simulink library "IOBlock_Library_TTC580"  (R2021a)
settings: Solver=ode45  StartTime=0.0  StopTime=10.0  RelTol=1e-3
PreLoadFcn:
  | addpath(genpath(fileparts(which('IOBlock_Library_TTC580'))));
  | %addpath(genpath(fileparts(which('IOBlock_Library_TTC580.mdl'))))
  | try
  | addpath(genpath([fileparts(which('IOBlock_Library_TTC580')),'\..\DBC_Importer']));
  | addpath(genpath([fileparts(which('IOBlock_Library_TTC580')),'\..\EEPROM_Importer']));
  | addpath(genpath([fileparts(which('IOBlock_Library_TTC580')),'\..\UserDoc']));
  | catch
  | warning('IOBlock_Library_TTC580: add path to DBC_Importer and EEPROM_Importer manually');
  | end
  | try
  | if exist('..\CustomPackage\scripts\OpenAllPackages.m','file')
  |      run('..\CustomPackage\scripts\OpenAllPackages.m'); %always available, ggf. empty
  | end
  | catch
  | warning('A problem occurred opening automatically the CustomPackage. Please open libraries manually');
  | end
  | try
  | set_param(0,'EditorSmartEditingHotParam','off');
  | catch
  | warning('Simlink preferences for ''Edit key parameter when adding new blocks'' needs to be unchecked manually');
  | end
undefined symbols (not defined in the file or in its folder): ADC_Absolute_10V, ADC_Absolute_32V, ADC_Absolute_5V, ADC_BoardTemp, ADC_ChannelInit, ADC_Current, ADC_Get, ADC_K15_, ADC_Ratiometric_10V, ADC_Ratiometric_5V, ADC_Resistive, ADC_SensorSupply, ADC_UBAT, bit_packing, bit_unpacking, CAN_ConfigMsg, compare2error, compare2FET_PROT_REENABLE, crc32_calc_intern, CRC32_EEPROM_Read, CRC32_EEPROM_Write, DIAG_EnterSafestate, DIAG_Status, DIAG_Status_internal, EEPROM_Mirror, EEPROM_Read, EEPROM_Read_OffsetIn, EEPROM_Read_Raw, EEPROM_Write, EEPROM_Write_OffsetIn, EEPROM_Write_Raw, EnterSafestate, FPU_Handler, Get_DI, Get_DI_VarThreshold, Get_K15_, Get_Pulse_Freq_Curr, Get_Pulse_Freq_Volt, Get_WakeUp, GetDateAndTime, IO_ADC_ResetProtection, IO_Blk_Lib_TTC500, IO_CAN_ReadMsg, IO_CAN_WriteMsg, IO_DI_Get, IO_DI_Init, IO_DI_Init_Var, IO_DO_GetCur, IO_DO_GetVoltage, IO_DO_Init, IO_DO_ResetProtection, IO_DO_Set, IO_Driver_GetSerialNumber, IO_Driver_GetVersionOfDriver, IO_Driver_GetVersionOfFPGA, IO_EEPROM_GetStatus, IO_EEPROM_Init, IO_EEPROM_Read_raw, IO_EEPROM_Write, IO_EEPROM_Write_OffsetIn ... (+73)
libraries: simulink x43
(part 7 of 18)

== system IOBlock_Library_TTC580/ADC Blocks TTC580 IOlib/ADC_Absolute_5V ==
  ADC_ChannelInit : Subsystem  LoadFcn=|  mask(ADC_ChannelInit_Code){SampleTime=-1, ttlib=IO_Blk_Lib_TTC500, ttDescription=ADC_ChannelInit, tt_iolib_version=0.19, adc_channel=adc_channel, adc_type=adc_type, range=range, pupd=pupd, sensor_supply=sensor_supply, safety_conf=NULL}
      | try
      | %
      | %Upgrade Information - standard BEGIN
      | new_color = 'blue';
      | new_ver = '0.19';
      | act_ver = get_param(gcb,'tt_iolib_version');
      | if not(strcmp(act_ver,new_ver))
      |     disp(['Upgrade block: ',gcb,char(10),'       Version: ',act_ver,' -> ',new_ver]);
      |     %switch - case for specific upgrade information e.g. additional parameter required 
      |     %Change appearance and version information
      |     set_param(gcb,'ForegroundColor',new_color);
      |     set_param(gcb,'tt_iolib_version',new_ver);
      | end
      | %Upgrade Information - standard END
      | catch
      | %Standard catch section BEGIN 
      | disp(' ');
      | disp('------------------------------------------------------------');
      | disp('An error occurred in a callback of the TTC580-BlockLib.');
      | disp(['Please check the parameters in the mask of ',gcb]);
      | disp('If you do not encounter any violations, then please '); 
      | disp('copy the following lines and report this to support@ttcontrol.com ');
      | disp('<< begin of error message dump >>');
      | disp(['Version of TTC580-BlockLib: ', get_param(gcb,'tt_iolib_version')]);
      | disp(get_param(gcb,'ttDescription'));
      | disp(gcb);
      | x=lasterror;disp(x.message);
      | disp(get_param(gcb,'MaskValues'));
      | disp(version);
      | disp(computer);
      | disp('<< end of error message dump >>');
      | disp('------------------------------------------------------------');
      | disp(' ');
      | %Standard catch section END
      | end
      mask help: Setup one ADC channel.
      mask init:
      | %
      settings: CopyFcn=%deleted
      mask Help: web(which('IO_ADC.h'))
      mask Callback adc_channel: %
      mask Callback adc_type: %
      mask Callback range: %
      mask Callback pupd: %
      mask Callback sensor_supply: %
      mask Callback safety_conf: %
  ADC_Get : Subsystem  LoadFcn=|  mask(ADC_Get_Code){SampleTime=-1, ttlib=IO_Blk_Lib_TTC500, ttDescription=ADC_Get, tt_iolib_version=0.19, adc_channel=adc_channel}
      | try
      | %
      | %Upgrade Information - standard BEGIN
      | new_color = 'blue';
      | new_ver = '0.19';
      | act_ver = get_param(gcb,'tt_iolib_version');
      | if not(strcmp(act_ver,new_ver))
      |     disp(['Upgrade block: ',gcb,char(10),'       Version: ',act_ver,' -> ',new_ver]);
      |     %switch - case for specific upgrade information e.g. additional parameter required 
      |     %Change appearance and version information
      |     set_param(gcb,'ForegroundColor',new_color);
      |     set_param(gcb,'tt_iolib_version',new_ver);
      | end
      | %Upgrade Information - standard END
      | catch
      | %Standard catch section BEGIN 
      | disp(' ');
      | disp('------------------------------------------------------------');
      | disp('An error occurred in a callback of the TTC580-BlockLib.');
      | disp(['Please check the parameters in the mask of ',gcb]);
      | disp('If you do not encounter any violations, then please '); 
      | disp('copy the following lines and report this to support@ttcontrol.com ');
      | disp('<< begin of error message dump >>');
      | disp(['Version of TTC580-BlockLib: ', get_param(gcb,'tt_iolib_version')]);
      | disp(get_param(gcb,'ttDescription'));
      | disp(gcb);
      | x=lasterror;disp(x.message);
      | disp(get_param(gcb,'MaskValues'));
      | disp(version);
      | disp(computer);
      | disp('<< end of error message dump >>');
      | disp('------------------------------------------------------------');
      | disp(' ');
      | %Standard catch section END
      | end
      mask help: Returns the value of the given ADC channel.
      mask init:
      | %
      settings: CopyFcn=%deleted
      mask Help: web(which('IO_ADC.h'))
      mask Callback adc_channel: %
  PWM_Init : Terminator
  PWM_Init1 : Terminator
  ErrorCode : Outport  VectorParamsAs1DForOutWhenUnconnected=off
  adc_value : Outport  Port=2  VectorParamsAs1DForOutWhenUnconnected=off
  wires:
  ADC_ChannelInit/1(ErrorCode) -> PWM_Init/1
  ADC_Get/3(fresh) -> PWM_Init1/1
  ADC_Get/1(ErrorCode) -> ErrorCode/1
  ADC_Get/2(adc_value) -> adc_value/1

== system IOBlock_Library_TTC580/ADC Blocks TTC580 IOlib/ADC_BoardTemp ==
  ADC_ChannelInit : Subsystem  LoadFcn=|  mask(ADC_ChannelInit_Code){SampleTime=-1, ttlib=IO_Blk_Lib_TTC500, ttDescription=ADC_ChannelInit, tt_iolib_version=0.19, adc_channel=adc_channel, adc_type=adc_type, range=range, pupd=pupd, sensor_supply=sensor_supply, safety_conf=NULL}
      | try
      | %
      | %Upgrade Information - standard BEGIN
      | new_color = 'blue';
      | new_ver = '0.19';
      | act_ver = get_param(gcb,'tt_iolib_version');
      | if not(strcmp(act_ver,new_ver))
      |     disp(['Upgrade block: ',gcb,char(10),'       Version: ',act_ver,' -> ',new_ver]);
      |     %switch - case for specific upgrade information e.g. additional parameter required 
      |     %Change appearance and version information
      |     set_param(gcb,'ForegroundColor',new_color);
      |     set_param(gcb,'tt_iolib_version',new_ver);
      | end
      | %Upgrade Information - standard END
      | catch
      | %Standard catch section BEGIN 
      | disp(' ');
      | disp('------------------------------------------------------------');
      | disp('An error occurred in a callback of the TTC580-BlockLib.');
      | disp(['Please check the parameters in the mask of ',gcb]);
      | disp('If you do not encounter any violations, then please '); 
      | disp('copy the following lines and report this to support@ttcontrol.com ');
      | disp('<< begin of error message dump >>');
      | disp(['Version of TTC580-BlockLib: ', get_param(gcb,'tt_iolib_version')]);
      | disp(get_param(gcb,'ttDescription'));
      | disp(gcb);
      | x=lasterror;disp(x.message);
      | disp(get_param(gcb,'MaskValues'));
      | disp(version);
      | disp(computer);
      | disp('<< end of error message dump >>');
      | disp('------------------------------------------------------------');
      | disp(' ');
      | %Standard catch section END
      | end
      mask help: Setup one ADC channel.
      mask init:
      | %
      settings: CopyFcn=%deleted
      mask Help: web(which('IO_ADC.h'))
      mask Callback adc_channel: %
      mask Callback adc_type: %
      mask Callback range: %
      mask Callback pupd: %
      mask Callback sensor_supply: %
      mask Callback safety_conf: %
  ADC_Get : Subsystem  LoadFcn=|  mask(ADC_Get_Code){SampleTime=-1, ttlib=IO_Blk_Lib_TTC500, ttDescription=ADC_Get, tt_iolib_version=0.19, adc_channel=adc_channel}
      | try
      | %
      | %Upgrade Information - standard BEGIN
      | new_color = 'blue';
      | new_ver = '0.19';
      | act_ver = get_param(gcb,'tt_iolib_version');
      | if not(strcmp(act_ver,new_ver))
      |     disp(['Upgrade block: ',gcb,char(10),'       Version: ',act_ver,' -> ',new_ver]);
      |     %switch - case for specific upgrade information e.g. additional parameter required 
      |     %Change appearance and version information
      |     set_param(gcb,'ForegroundColor',new_color);
      |     set_param(gcb,'tt_iolib_version',new_ver);
      | end
      | %Upgrade Information - standard END
      | catch
      | %Standard catch section BEGIN 
      | disp(' ');
      | disp('------------------------------------------------------------');
      | disp('An error occurred in a callback of the TTC580-BlockLib.');
      | disp(['Please check the parameters in the mask of ',gcb]);
      | disp('If you do not encounter any violations, then please '); 
      | disp('copy the following lines and report this to support@ttcontrol.com ');
      | disp('<< begin of error message dump >>');
      | disp(['Version of TTC580-BlockLib: ', get_param(gcb,'tt_iolib_version')]);
      | disp(get_param(gcb,'ttDescription'));
      | disp(gcb);
      | x=lasterror;disp(x.message);
      | disp(get_param(gcb,'MaskValues'));
      | disp(version);
      | disp(computer);
      | disp('<< end of error message dump >>');
      | disp('------------------------------------------------------------');
      | disp(' ');
      | %Standard catch section END
      | end
      mask help: Returns the value of the given ADC channel.
      mask init:
      | %
      settings: CopyFcn=%deleted
      mask Help: web(which('IO_ADC.h'))
      mask Callback adc_channel: %
  Add : Sum  Inputs=+-
  Constant : Constant  Value=10000  OutDataTypeStr=int32
  Constant1 : Constant  Value=100  OutDataTypeStr=int32
  Data Type Conversion : DataTypeConversion  OutDataTypeStr=int32
  Divide : Product  Inputs=*/
  PWM_Init : Terminator
  PWM_Init1 : Terminator
  ErrorCode : Outport  VectorParamsAs1DForOutWhenUnconnected=off
  Temperature : Outport  Port=2  VectorParamsAs1DForOutWhenUnconnected=off
  wires:
  ADC_ChannelInit/1(ErrorCode) -> PWM_Init/1
  ADC_Get/3(fresh) -> PWM_Init1/1
  ADC_Get/1(ErrorCode) -> ErrorCode/1
  ADC_Get/2(adc_value) -> Data Type Conversion/1
  Data Type Conversion/1 -> Add/1
  Constant/1 -> Add/2
  Add/1 -> Divide/1
  Constant1/1 -> Divide/2
  Divide/1 -> Temperature/1

== system IOBlock_Library_TTC580/ADC Blocks TTC580 IOlib/ADC_Current ==
  ADC_ChannelInit : Subsystem  LoadFcn=|  mask(ADC_ChannelInit_Code){SampleTime=-1, ttlib=IO_Blk_Lib_TTC500, ttDescription=ADC_ChannelInit, tt_iolib_version=0.19, adc_channel=adc_channel, adc_type=adc_type, range=range, pupd=pupd, sensor_supply=sensor_supply, safety_conf=NULL}
      | try
      | %
      | %Upgrade Information - standard BEGIN
      | new_color = 'blue';
      | new_ver = '0.19';
      | act_ver = get_param(gcb,'tt_iolib_version');
      | if not(strcmp(act_ver,new_ver))
      |     disp(['Upgrade block: ',gcb,char(10),'       Version: ',act_ver,' -> ',new_ver]);
      |     %switch - case for specific upgrade information e.g. additional parameter required 
      |     %Change appearance and version information
      |     set_param(gcb,'ForegroundColor',new_color);
      |     set_param(gcb,'tt_iolib_version',new_ver);
      | end
      | %Upgrade Information - standard END
      | catch
      | %Standard catch section BEGIN 
      | disp(' ');
      | disp('------------------------------------------------------------');
      | disp('An error occurred in a callback of the TTC580-BlockLib.');
      | disp(['Please check the parameters in the mask of ',gcb]);
      | disp('If you do not encounter any violations, then please '); 
      | disp('copy the following lines and report this to support@ttcontrol.com ');
      | disp('<< begin of error message dump >>');
      | disp(['Version of TTC580-BlockLib: ', get_param(gcb,'tt_iolib_version')]);
      | disp(get_param(gcb,'ttDescription'));
      | disp(gcb);
      | x=lasterror;disp(x.message);
      | disp(get_param(gcb,'MaskValues'));
      | disp(version);
      | disp(computer);
      | disp('<< end of error message dump >>');
      | disp('------------------------------------------------------------');
      | disp(' ');
      | %Standard catch section END
      | end
      mask help: Setup one ADC channel.
      mask init:
      | %
      settings: CopyFcn=%deleted
      mask Help: web(which('IO_ADC.h'))
      mask Callback adc_channel: %
      mask Callback adc_type: %
      mask Callback range: %
      mask Callback pupd: %
      mask Callback sensor_supply: %
      mask Callback safety_conf: %
  ADC_Get : Subsystem  LoadFcn=|  mask(ADC_Get_Code){SampleTime=-1, ttlib=IO_Blk_Lib_TTC500, ttDescription=ADC_Get, tt_iolib_version=0.19, adc_channel=adc_channel}
      | try
      | %
      | %Upgrade Information - standard BEGIN
      | new_color = 'blue';
      | new_ver = '0.19';
      | act_ver = get_param(gcb,'tt_iolib_version');
      | if not(strcmp(act_ver,new_ver))
      |     disp(['Upgrade block: ',gcb,char(10),'       Version: ',act_ver,' -> ',new_ver]);
      |     %switch - case for specific upgrade information e.g. additional parameter required 
      |     %Change appearance and version information
      |     set_param(gcb,'ForegroundColor',new_color);
      |     set_param(gcb,'tt_iolib_version',new_ver);
      | end
      | %Upgrade Information - standard END
      | catch
      | %Standard catch section BEGIN 
      | disp(' ');
      | disp('------------------------------------------------------------');
      | disp('An error occurred in a callback of the TTC580-BlockLib.');
      | disp(['Please check the parameters in the mask of ',gcb]);
      | disp('If you do not encounter any violations, then please '); 
      | disp('copy the following lines and report this to support@ttcontrol.com ');
      | disp('<< begin of error message dump >>');
      | disp(['Version of TTC580-BlockLib: ', get_param(gcb,'tt_iolib_version')]);
      | disp(get_param(gcb,'ttDescription'));
      | disp(gcb);
      | x=lasterror;disp(x.message);
      | disp(get_param(gcb,'MaskValues'));
      | disp(version);
      | disp(computer);
      | disp('<< end of error message dump >>');
      | disp('------------------------------------------------------------');
      | disp(' ');
      | %Standard catch section END
      | end
      mask help: Returns the value of the given ADC channel.
      mask init:
      | %
      settings: CopyFcn=%deleted
      mask Help: web(which('IO_ADC.h'))
      mask Callback adc_channel: %
  IO_ADC_ResetProtection : Subsystem  LoadFcn=|  mask(IO_ADC_ResetProtection_Code){SampleTime=-1, ttlib=IO_Blk_Lib_TTC500, ttDescription=IO_ADC_ResetProtection, tt_iolib_version=0.19, adc_channel=adc_channel}
      | try
      | %
      | %Upgrade Information - standard BEGIN
      | new_color = 'blue';
      | new_ver = '0.19';
      | act_ver = get_param(gcb,'tt_iolib_version');
      | if not(strcmp(act_ver,new_ver))
      |     disp(['Upgrade block: ',gcb,char(10),'       Version: ',act_ver,' -> ',new_ver]);
      |     %switch - case for specific upgrade information e.g. additional parameter required 
      |     %Change appearance and version information
      |     set_param(gcb,'ForegroundColor',new_color);
      |     set_param(gcb,'tt_iolib_version',new_ver);
      | end
      | %Upgrade Information - standard END
      | catch
      | %Standard catch section BEGIN 
      | disp(' ');
      | disp('------------------------------------------------------------');
      | disp('An error occurred in a callback of the TTC580-BlockLib.');
      | disp(['Please check the parameters in the mask of ',gcb]);
      | disp('If you do not encounter any violations, then please '); 
      | disp('copy the following lines and report this to support@ttcontrol.com ');
      | disp('<< begin of error message dump >>');
      | disp(['Version of TTC580-BlockLib: ', get_param(gcb,'tt_iolib_version')]);
      | disp(get_param(gcb,'ttDescription'));
      | disp(gcb);
      | x=lasterror;disp(x.message);
      | disp(get_param(gcb,'MaskValues'));
      | disp(version);
      | disp(computer);
      | disp('<< end of error message dump >>');
      | disp('------------------------------------------------------------');
      | disp(' ');
      | %Standard catch section END
      | end
      mask help: Reset the FET protection for an ADC channel.
      mask init:
      | %
      settings: CopyFcn=%deleted
      mask Help: web(which('IO_ADC.h'))
      mask Callback adc_channel: %
  PWM_Init : Terminator
  PWM_Init1 : Terminator
  Terminator1 : Terminator
  Terminator3 : Terminator
  compare2FET_PROT_REENABLE : Subsystem  LoadFcn=|  mask(compare2FET_PROT_REENABLE_Code){SampleTime=-1, ttlib=IO_Blk_Lib_TTC500, ttDescription=compare2FET_PROT_REENABLE, tt_iolib_version=0.19, define=IO_E_FET_PROT_REENABLE}
      | try
      | %
      | %Upgrade Information - standard BEGIN
      | new_color = 'blue';
      | new_ver = '0.19';
      | act_ver = get_param(gcb,'tt_iolib_version');
      | if not(strcmp(act_ver,new_ver))
      |     disp(['Upgrade block: ',gcb,char(10),'       Version: ',act_ver,' -> ',new_ver]);
      |     %switch - case for specific upgrade information e.g. additional parameter required 
      |     %Change appearance and version information
      |     set_param(gcb,'ForegroundColor',new_color);
      |     set_param(gcb,'tt_iolib_version',new_ver);
      | end
      | %Upgrade Information - standard END
      | catch
      | %Standard catch section BEGIN 
      | disp(' ');
      | disp('------------------------------------------------------------');
      | disp('An error occurred in a callback of the TTC580-BlockLib.');
      | disp(['Please check the parameters in the mask of ',gcb]);
      | disp('If you do not encounter any violations, then please '); 
      | disp('copy the following lines and report this to support@ttcontrol.com ');
      | disp('<< begin of error message dump >>');
      | disp(['Version of TTC580-BlockLib: ', get_param(gcb,'tt_iolib_version')]);
      | disp(get_param(gcb,'ttDescription'));
      | disp(gcb);
      | x=lasterror;disp(x.message);
      | disp(get_param(gcb,'MaskValues'));
      | disp(version);
      | disp(computer);
      | disp('<< end of error message dump >>');
      | disp('------------------------------------------------------------');
      | disp(' ');
      | %Standard catch section END
      | end
      mask help: The ErrorCode that is output from an I/O-Block is compared against IO_E_FET_PROT_REENABLE.
      mask init:
      | %
      settings: CopyFcn=%deleted
      mask Help: web(which('~.h'))
      mask Callback define: %
  ErrorCode : Outport  VectorParamsAs1DForOutWhenUnconnected=off
  adc_value : Outport  Port=2  VectorParamsAs1DForOutWhenUnconnected=off
  wires:
  ADC_ChannelInit/1(ErrorCode) -> PWM_Init/1
  ADC_Get/3(fresh) -> PWM_Init1/1
  ADC_Get/1(ErrorCode) -> ErrorCode/1, compare2FET_PROT_REENABLE/1(Errorcode)
  ADC_Get/2(adc_value) -> adc_value/1
  IO_ADC_ResetProtection/1(ErrorCode) -> Terminator3/1
  IO_ADC_ResetProtection/2(reset_cnt) -> Terminator1/1
  compare2FET_PROT_REENABLE/1(b_compare) -> IO_ADC_ResetProtection/Trigger

== system IOBlock_Library_TTC580/ADC Blocks TTC580 IOlib/ADC_K15_ ==
  ADC_ChannelInit : Subsystem  LoadFcn=|  mask(ADC_ChannelInit_Code){SampleTime=-1, ttlib=IO_Blk_Lib_TTC500, ttDescription=ADC_ChannelInit, tt_iolib_version=0.19, adc_channel=adc_channel, adc_type=adc_type, range=range, pupd=pupd, sensor_supply=sensor_supply, safety_conf=NULL}
      | try
      | %
      | %Upgrade Information - standard BEGIN
      | new_color = 'blue';
      | new_ver = '0.19';
      | act_ver = get_param(gcb,'tt_iolib_version');
      | if not(strcmp(act_ver,new_ver))
      |     disp(['Upgrade block: ',gcb,char(10),'       Version: ',act_ver,' -> ',new_ver]);
      |     %switch - case for specific upgrade information e.g. additional parameter required 
      |     %Change appearance and version information
      |     set_param(gcb,'ForegroundColor',new_color);
      |     set_param(gcb,'tt_iolib_version',new_ver);
      | end
      | %Upgrade Information - standard END
      | catch
      | %Standard catch section BEGIN 
      | disp(' ');
      | disp('------------------------------------------------------------');
      | disp('An error occurred in a callback of the TTC580-BlockLib.');
      | disp(['Please check the parameters in the mask of ',gcb]);
      | disp('If you do not encounter any violations, then please '); 
      | disp('copy the following lines and report this to support@ttcontrol.com ');
      | disp('<< begin of error message dump >>');
      | disp(['Version of TTC580-BlockLib: ', get_param(gcb,'tt_iolib_version')]);
      | disp(get_param(gcb,'ttDescription'));
      | disp(gcb);
      | x=lasterror;disp(x.message);
      | disp(get_param(gcb,'MaskValues'));
      | disp(version);
      | disp(computer);
      | disp('<< end of error message dump >>');
      | disp('------------------------------------------------------------');
      | disp(' ');
      | %Standard catch section END
      | end
      mask help: Setup one ADC channel.
      mask init:
      | %
      settings: CopyFcn=%deleted
      mask Help: web(which('IO_ADC.h'))
      mask Callback adc_channel: %
      mask Callback adc_type: %
      mask Callback range: %
      mask Callback pupd: %
      mask Callback sensor_supply: %
      mask Callback safety_conf: %
  ADC_Get : Subsystem  LoadFcn=|  mask(ADC_Get_Code){SampleTime=-1, ttlib=IO_Blk_Lib_TTC500, ttDescription=ADC_Get, tt_iolib_version=0.19, adc_channel=adc_channel}
      | try
      | %
      | %Upgrade Information - standard BEGIN
      | new_color = 'blue';
      | new_ver = '0.19';
      | act_ver = get_param(gcb,'tt_iolib_version');
      | if not(strcmp(act_ver,new_ver))
      |     disp(['Upgrade block: ',gcb,char(10),'       Version: ',act_ver,' -> ',new_ver]);
      |     %switch - case for specific upgrade information e.g. additional parameter required 
      |     %Change appearance and version information
      |     set_param(gcb,'ForegroundColor',new_color);
      |     set_param(gcb,'tt_iolib_version',new_ver);
      | end
      | %Upgrade Information - standard END
      | catch
      | %Standard catch section BEGIN 
      | disp(' ');
      | disp('------------------------------------------------------------');
      | disp('An error occurred in a callback of the TTC580-BlockLib.');
      | disp(['Please check the parameters in the mask of ',gcb]);
      | disp('If you do not encounter any violations, then please '); 
      | disp('copy the following lines and report this to support@ttcontrol.com ');
      | disp('<< begin of error message dump >>');
      | disp(['Version of TTC580-BlockLib: ', get_param(gcb,'tt_iolib_version')]);
      | disp(get_param(gcb,'ttDescription'));
      | disp(gcb);
      | x=lasterror;disp(x.message);
      | disp(get_param(gcb,'MaskValues'));
      | disp(version);
      | disp(computer);
      | disp('<< end of error message dump >>');
      | disp('------------------------------------------------------------');
      | disp(' ');
      | %Standard catch section END
      | end
      mask help: Returns the value of the given ADC channel.
      mask init:
      | %
      settings: CopyFcn=%deleted
      mask Help: web(which('IO_ADC.h'))
      mask Callback adc_channel: %
  PWM_Init : Terminator
  PWM_Init1 : Terminator
  ErrorCode : Outport  VectorParamsAs1DForOutWhenUnconnected=off
  adc_value : Outport  Port=2  VectorParamsAs1DForOutWhenUnconnected=off
  wires:
  ADC_Get/3(fresh) -> PWM_Init1/1
  ADC_Get/2(adc_value) -> adc_value/1
  ADC_Get/1(ErrorCode) -> ErrorCode/1
  ADC_ChannelInit/1(ErrorCode) -> PWM_Init/1

== system IOBlock_Library_TTC580/ADC Blocks TTC580 IOlib/ADC_Ratiometric_10V ==
  ADC_ChannelInit : Subsystem  LoadFcn=|  mask(ADC_ChannelInit_Code){SampleTime=-1, ttlib=IO_Blk_Lib_TTC500, ttDescription=ADC_ChannelInit, tt_iolib_version=0.19, adc_channel=adc_channel, adc_type=adc_type, range=range, pupd=pupd, sensor_supply=sensor_supply, safety_conf=NULL}
      | try
      | %
      | %Upgrade Information - standard BEGIN
      | new_color = 'blue';
      | new_ver = '0.19';
      | act_ver = get_param(gcb,'tt_iolib_version');
      | if not(strcmp(act_ver,new_ver))
      |     disp(['Upgrade block: ',gcb,char(10),'       Version: ',act_ver,' -> ',new_ver]);
      |     %switch - case for specific upgrade information e.g. additional parameter required 
      |     %Change appearance and version information
      |     set_param(gcb,'ForegroundColor',new_color);
      |     set_param(gcb,'tt_iolib_version',new_ver);
      | end
      | %Upgrade Information - standard END
      | catch
      | %Standard catch section BEGIN 
      | disp(' ');
      | disp('------------------------------------------------------------');
      | disp('An error occurred in a callback of the TTC580-BlockLib.');
      | disp(['Please check the parameters in the mask of ',gcb]);
      | disp('If you do not encounter any violations, then please '); 
      | disp('copy the following lines and report this to support@ttcontrol.com ');
      | disp('<< begin of error message dump >>');
      | disp(['Version of TTC580-BlockLib: ', get_param(gcb,'tt_iolib_version')]);
      | disp(get_param(gcb,'ttDescription'));
      | disp(gcb);
      | x=lasterror;disp(x.message);
      | disp(get_param(gcb,'MaskValues'));
      | disp(version);
      | disp(computer);
      | disp('<< end of error message dump >>');
      | disp('------------------------------------------------------------');
      | disp(' ');
      | %Standard catch section END
      | end
      mask help: Setup one ADC channel.
      mask init:
      | %
      settings: CopyFcn=%deleted
      mask Help: web(which('IO_ADC.h'))
      mask Callback adc_channel: %
      mask Callback adc_type: %
      mask Callback range: %
      mask Callback pupd: %
      mask Callback sensor_supply: %
      mask Callback safety_conf: %
  ADC_Get : Subsystem  LoadFcn=|  mask(ADC_Get_Code){SampleTime=-1, ttlib=IO_Blk_Lib_TTC500, ttDescription=ADC_Get, tt_iolib_version=0.19, adc_channel=adc_channel}
      | try
      | %
      | %Upgrade Information - standard BEGIN
      | new_color = 'blue';
      | new_ver = '0.19';
      | act_ver = get_param(gcb,'tt_iolib_version');
      | if not(strcmp(act_ver,new_ver))
      |     disp(['Upgrade block: ',gcb,char(10),'       Version: ',act_ver,' -> ',new_ver]);
      |     %switch - case for specific upgrade information e.g. additional parameter required 
      |     %Change appearance and version information
      |     set_param(gcb,'ForegroundColor',new_color);
      |     set_param(gcb,'tt_iolib_version',new_ver);
      | end
      | %Upgrade Information - standard END
      | catch
      | %Standard catch section BEGIN 
      | disp(' ');
      | disp('------------------------------------------------------------');
      | disp('An error occurred in a callback of the TTC580-BlockLib.');
      | disp(['Please check the parameters in the mask of ',gcb]);
      | disp('If you do not encounter any violations, then please '); 
      | disp('copy the following lines and report this to support@ttcontrol.com ');
      | disp('<< begin of error message dump >>');
      | disp(['Version of TTC580-BlockLib: ', get_param(gcb,'tt_iolib_version')]);
      | disp(get_param(gcb,'ttDescription'));
      | disp(gcb);
      | x=lasterror;disp(x.message);
      | disp(get_param(gcb,'MaskValues'));
      | disp(version);
      | disp(computer);
      | disp('<< end of error message dump >>');
      | disp('------------------------------------------------------------');
      | disp(' ');
      | %Standard catch section END
      | end
      mask help: Returns the value of the given ADC channel.
      mask init:
      | %
      settings: CopyFcn=%deleted
      mask Help: web(which('IO_ADC.h'))
      mask Callback adc_channel: %
  POWER_Set_Init : Subsystem  LoadFcn=|  mask(POWER_Set_Init_Code){SampleTime=-1, ttlib=IO_Blk_Lib_TTC500, ttDescription=POWER_Set_Init, tt_iolib_version=0.19, pin=sensor_supply, mode=volt_sensor_supply}
      | try
      | %
      | %Upgrade Information - standard BEGIN
      | new_color = 'blue';
      | new_ver = '0.19';
      | act_ver = get_param(gcb,'tt_iolib_version');
      | if not(strcmp(act_ver,new_ver))
      |     disp(['Upgrade block: ',gcb,char(10),'       Version: ',act_ver,' -> ',new_ver]);
      |     %switch - case for specific upgrade information e.g. additional parameter required 
      |     %Change appearance and version information
      |     set_param(gcb,'ForegroundColor',new_color);
      |     set_param(gcb,'tt_iolib_version',new_ver);
      | end
      | %Upgrade Information - standard END
      | catch
      | %Standard catch section BEGIN 
      | disp(' ');
      | disp('------------------------------------------------------------');
      | disp('An error occurred in a callback of the TTC580-BlockLib.');
      | disp(['Please check the parameters in the mask of ',gcb]);
      | disp('If you do not encounter any violations, then please '); 
      | disp('copy the following lines and report this to support@ttcontrol.com ');
      | disp('<< begin of error message dump >>');
      | disp(['Version of TTC580-BlockLib: ', get_param(gcb,'tt_iolib_version')]);
      | disp(get_param(gcb,'ttDescription'));
      | disp(gcb);
      | x=lasterror;disp(x.message);
      | disp(get_param(gcb,'MaskValues'));
      | disp(version);
      | disp(computer);
      | disp('<< end of error message dump >>');
      | disp('------------------------------------------------------------');
      | disp(' ');
      | %Standard catch section END
      | end
      mask help: Sets a certain mode of the Power IC.
      mask init:
      | %
      settings: CopyFcn=%deleted
      mask Help: web(which('IO_POWER.h'))
      mask Callback pin: %
      mask Callback mode: %
  PWM_Init : Terminator
  PWM_Init1 : Terminator
  PWM_Init2 : Terminator
  ErrorCode : Outport  VectorParamsAs1DForOutWhenUnconnected=off
  adc_value : Outport  Port=2  VectorParamsAs1DForOutWhenUnconnected=off
  wires:
  ADC_ChannelInit/1(ErrorCode) -> PWM_Init/1
  ADC_Get/3(fresh) -> PWM_Init1/1
  ADC_Get/1(ErrorCode) -> ErrorCode/1
  ADC_Get/2(adc_value) -> adc_value/1
  POWER_Set_Init/1(ErrorCode) -> PWM_Init2/1

== system IOBlock_Library_TTC580/ADC Blocks TTC580 IOlib/ADC_Ratiometric_5V ==
  ADC_ChannelInit : Subsystem  LoadFcn=|  mask(ADC_ChannelInit_Code){SampleTime=-1, ttlib=IO_Blk_Lib_TTC500, ttDescription=ADC_ChannelInit, tt_iolib_version=0.19, adc_channel=adc_channel, adc_type=adc_type, range=range, pupd=pupd, sensor_supply=sensor_supply, safety_conf=NULL}
      | try
      | %
      | %Upgrade Information - standard BEGIN
      | new_color = 'blue';
      | new_ver = '0.19';
      | act_ver = get_param(gcb,'tt_iolib_version');
      | if not(strcmp(act_ver,new_ver))
      |     disp(['Upgrade block: ',gcb,char(10),'       Version: ',act_ver,' -> ',new_ver]);
      |     %switch - case for specific upgrade information e.g. additional parameter required 
      |     %Change appearance and version information
      |     set_param(gcb,'ForegroundColor',new_color);
      |     set_param(gcb,'tt_iolib_version',new_ver);
      | end
      | %Upgrade Information - standard END
      | catch
      | %Standard catch section BEGIN 
      | disp(' ');
      | disp('------------------------------------------------------------');
      | disp('An error occurred in a callback of the TTC580-BlockLib.');
      | disp(['Please check the parameters in the mask of ',gcb]);
      | disp('If you do not encounter any violations, then please '); 
      | disp('copy the following lines and report this to support@ttcontrol.com ');
      | disp('<< begin of error message dump >>');
      | disp(['Version of TTC580-BlockLib: ', get_param(gcb,'tt_iolib_version')]);
      | disp(get_param(gcb,'ttDescription'));
      | disp(gcb);
      | x=lasterror;disp(x.message);
      | disp(get_param(gcb,'MaskValues'));
      | disp(version);
      | disp(computer);
      | disp('<< end of error message dump >>');
      | disp('------------------------------------------------------------');
      | disp(' ');
      | %Standard catch section END
      | end
      mask help: Setup one ADC channel.
      mask init:
      | %
      settings: CopyFcn=%deleted
      mask Help: web(which('IO_ADC.h'))
      mask Callback adc_channel: %
      mask Callback adc_type: %
      mask Callback range: %
      mask Callback pupd: %
      mask Callback sensor_supply: %
      mask Callback safety_conf: %
  ADC_Get : Subsystem  LoadFcn=|  mask(ADC_Get_Code){SampleTime=-1, ttlib=IO_Blk_Lib_TTC500, ttDescription=ADC_Get, tt_iolib_version=0.19, adc_channel=adc_channel}
      | try
      | %
      | %Upgrade Information - standard BEGIN
      | new_color = 'blue';
      | new_ver = '0.19';
      | act_ver = get_param(gcb,'tt_iolib_version');
      | if not(strcmp(act_ver,new_ver))
      |     disp(['Upgrade block: ',gcb,char(10),'       Version: ',act_ver,' -> ',new_ver]);
      |     %switch - case for specific upgrade information e.g. additional parameter required 
      |     %Change appearance and version information
      |     set_param(gcb,'ForegroundColor',new_color);
      |     set_param(gcb,'tt_iolib_version',new_ver);
      | end
      | %Upgrade Information - standard END
      | catch
      | %Standard catch section BEGIN 
      | disp(' ');
      | disp('------------------------------------------------------------');
      | disp('An error occurred in a callback of the TTC580-BlockLib.');
      | disp(['Please check the parameters in the mask of ',gcb]);
      | disp('If you do not encounter any violations, then please '); 
      | disp('copy the following lines and report this to support@ttcontrol.com ');
      | disp('<< begin of error message dump >>');
      | disp(['Version of TTC580-BlockLib: ', get_param(gcb,'tt_iolib_version')]);
      | disp(get_param(gcb,'ttDescription'));
      | disp(gcb);
      | x=lasterror;disp(x.message);
      | disp(get_param(gcb,'MaskValues'));
      | disp(version);
      | disp(computer);
      | disp('<< end of error message dump >>');
      | disp('------------------------------------------------------------');
      | disp(' ');
      | %Standard catch section END
      | end
      mask help: Returns the value of the given ADC channel.
      mask init:
      | %
      settings: CopyFcn=%deleted
      mask Help: web(which('IO_ADC.h'))
      mask Callback adc_channel: %
  POWER_Set_Init : Subsystem  LoadFcn=|  mask(POWER_Set_Init_Code){SampleTime=-1, ttlib=IO_Blk_Lib_TTC500, ttDescription=POWER_Set_Init, tt_iolib_version=0.19, pin=sensor_supply, mode=volt_sensor_supply}
      | try
      | %
      | %Upgrade Information - standard BEGIN
      | new_color = 'blue';
      | new_ver = '0.19';
      | act_ver = get_param(gcb,'tt_iolib_version');
      | if not(strcmp(act_ver,new_ver))
      |     disp(['Upgrade block: ',gcb,char(10),'       Version: ',act_ver,' -> ',new_ver]);
      |     %switch - case for specific upgrade information e.g. additional parameter required 
      |     %Change appearance and version information
      |     set_param(gcb,'ForegroundColor',new_color);
      |     set_param(gcb,'tt_iolib_version',new_ver);
      | end
      | %Upgrade Information - standard END
      | catch
      | %Standard catch section BEGIN 
      | disp(' ');
      | disp('------------------------------------------------------------');
      | disp('An error occurred in a callback of the TTC580-BlockLib.');
      | disp(['Please check the parameters in the mask of ',gcb]);
      | disp('If you do not encounter any violations, then please '); 
      | disp('copy the following lines and report this to support@ttcontrol.com ');
      | disp('<< begin of error message dump >>');
      | disp(['Version of TTC580-BlockLib: ', get_param(gcb,'tt_iolib_version')]);
      | disp(get_param(gcb,'ttDescription'));
      | disp(gcb);
      | x=lasterror;disp(x.message);
      | disp(get_param(gcb,'MaskValues'));
      | disp(version);
      | disp(computer);
      | disp('<< end of error message dump >>');
      | disp('------------------------------------------------------------');
      | disp(' ');
      | %Standard catch section END
      | end
      mask help: Sets a certain mode of the Power IC.
      mask init:
      | %
      settings: CopyFcn=%deleted
      mask Help: web(which('IO_POWER.h'))
      mask Callback pin: %
      mask Callback mode: %
  PWM_Init : Terminator
  PWM_Init1 : Terminator
  PWM_Init2 : Terminator
  ErrorCode : Outport  VectorParamsAs1DForOutWhenUnconnected=off
  adc_value : Outport  Port=2  VectorParamsAs1DForOutWhenUnconnected=off
  wires:
  POWER_Set_Init/1(ErrorCode) -> PWM_Init2/1
  ADC_Get/2(adc_value) -> adc_value/1
  ADC_Get/1(ErrorCode) -> ErrorCode/1
  ADC_Get/3(fresh) -> PWM_Init1/1
  ADC_ChannelInit/1(ErrorCode) -> PWM_Init/1

== system IOBlock_Library_TTC580/ADC Blocks TTC580 IOlib/ADC_Resistive ==
  ADC_ChannelInit : Subsystem  LoadFcn=|  mask(ADC_ChannelInit_Code){SampleTime=-1, ttlib=IO_Blk_Lib_TTC500, ttDescription=ADC_ChannelInit, tt_iolib_version=0.19, adc_channel=adc_channel, adc_type=adc_type, range=range, pupd=pupd, sensor_supply=sensor_supply, safety_conf=NULL}
      | try
      | %
      | %Upgrade Information - standard BEGIN
      | new_color = 'blue';
      | new_ver = '0.19';
      | act_ver = get_param(gcb,'tt_iolib_version');
      | if not(strcmp(act_ver,new_ver))
      |     disp(['Upgrade block: ',gcb,char(10),'       Version: ',act_ver,' -> ',new_ver]);
      |     %switch - case for specific upgrade information e.g. additional parameter required 
      |     %Change appearance and version information
      |     set_param(gcb,'ForegroundColor',new_color);
      |     set_param(gcb,'tt_iolib_version',new_ver);
      | end
      | %Upgrade Information - standard END
      | catch
      | %Standard catch section BEGIN 
      | disp(' ');
      | disp('------------------------------------------------------------');
      | disp('An error occurred in a callback of the TTC580-BlockLib.');
      | disp(['Please check the parameters in the mask of ',gcb]);
      | disp('If you do not encounter any violations, then please '); 
      | disp('copy the following lines and report this to support@ttcontrol.com ');
      | disp('<< begin of error message dump >>');
      | disp(['Version of TTC580-BlockLib: ', get_param(gcb,'tt_iolib_version')]);
      | disp(get_param(gcb,'ttDescription'));
      | disp(gcb);
      | x=lasterror;disp(x.message);
      | disp(get_param(gcb,'MaskValues'));
      | disp(version);
      | disp(computer);
      | disp('<< end of error message dump >>');
      | disp('------------------------------------------------------------');
      | disp(' ');
      | %Standard catch section END
      | end
      mask help: Setup one ADC channel.
      mask init:
      | %
      settings: CopyFcn=%deleted
      mask Help: web(which('IO_ADC.h'))
      mask Callback adc_channel: %
      mask Callback adc_type: %
      mask Callback range: %
      mask Callback pupd: %
      mask Callback sensor_supply: %
      mask Callback safety_conf: %
  ADC_Get : Subsystem  LoadFcn=|  mask(ADC_Get_Code){SampleTime=-1, ttlib=IO_Blk_Lib_TTC500, ttDescription=ADC_Get, tt_iolib_version=0.19, adc_channel=adc_channel}
      | try
      | %
      | %Upgrade Information - standard BEGIN
      | new_color = 'blue';
      | new_ver = '0.19';
      | act_ver = get_param(gcb,'tt_iolib_version');
      | if not(strcmp(act_ver,new_ver))
      |     disp(['Upgrade block: ',gcb,char(10),'       Version: ',act_ver,' -> ',new_ver]);
      |     %switch - case for specific upgrade information e.g. additional parameter required 
      |     %Change appearance and version information
      |     set_param(gcb,'ForegroundColor',new_color);
      |     set_param(gcb,'tt_iolib_version',new_ver);
      | end
      | %Upgrade Information - standard END
      | catch
      | %Standard catch section BEGIN 
      | disp(' ');
      | disp('------------------------------------------------------------');
      | disp('An error occurred in a callback of the TTC580-BlockLib.');
      | disp(['Please check the parameters in the mask of ',gcb]);
      | disp('If you do not encounter any violations, then please '); 
      | disp('copy the following lines and report this to support@ttcontrol.com ');
      | disp('<< begin of error message dump >>');
      | disp(['Version of TTC580-BlockLib: ', get_param(gcb,'tt_iolib_version')]);
      | disp(get_param(gcb,'ttDescription'));
      | disp(gcb);
      | x=lasterror;disp(x.message);
      | disp(get_param(gcb,'MaskValues'));
      | disp(version);
      | disp(computer);
      | disp('<< end of error message dump >>');
      | disp('------------------------------------------------------------');
      | disp(' ');
      | %Standard catch section END
      | end
      mask help: Returns the value of the given ADC channel.
      mask init:
      | %
      settings: CopyFcn=%deleted
      mask Help: web(which('IO_ADC.h'))
      mask Callback adc_channel: %
  PWM_Init : Terminator
  PWM_Init1 : Terminator
  ErrorCode : Outport  VectorParamsAs1DForOutWhenUnconnected=off
  adc_value : Outport  Port=2  VectorParamsAs1DForOutWhenUnconnected=off
  wires:
  ADC_ChannelInit/1(ErrorCode) -> PWM_Init/1
  ADC_Get/3(fresh) -> PWM_Init1/1
  ADC_Get/1(ErrorCode) -> ErrorCode/1
  ADC_Get/2(adc_value) -> adc_value/1

== system IOBlock_Library_TTC580/ADC Blocks TTC580 IOlib/ADC_SensorSupply ==
  ADC_ChannelInit : Subsystem  LoadFcn=|  mask(ADC_ChannelInit_Code){SampleTime=-1, ttlib=IO_Blk_Lib_TTC500, ttDescription=ADC_ChannelInit, tt_iolib_version=0.19, adc_channel=adc_channel, adc_type=adc_type, range=range, pupd=pupd, sensor_supply=sensor_supply, safety_conf=NULL}
      | try
      | %
      | %Upgrade Information - standard BEGIN
      | new_color = 'blue';
      | new_ver = '0.19';
      | act_ver = get_param(gcb,'tt_iolib_version');
      | if not(strcmp(act_ver,new_ver))
      |     disp(['Upgrade block: ',gcb,char(10),'       Version: ',act_ver,' -> ',new_ver]);
      |     %switch - case for specific upgrade information e.g. additional parameter required 
      |     %Change appearance and version information
      |     set_param(gcb,'ForegroundColor',new_color);
      |     set_param(gcb,'tt_iolib_version',new_ver);
      | end
      | %Upgrade Information - standard END
      | catch
      | %Standard catch section BEGIN 
      | disp(' ');
      | disp('------------------------------------------------------------');
      | disp('An error occurred in a callback of the TTC580-BlockLib.');
      | disp(['Please check the parameters in the mask of ',gcb]);
      | disp('If you do not encounter any violations, then please '); 
      | disp('copy the following lines and report this to support@ttcontrol.com ');
      | disp('<< begin of error message dump >>');
      | disp(['Version of TTC580-BlockLib: ', get_param(gcb,'tt_iolib_version')]);
      | disp(get_param(gcb,'ttDescription'));
      | disp(gcb);
      | x=lasterror;disp(x.message);
      | disp(get_param(gcb,'MaskValues'));
      | disp(version);
      | disp(computer);
      | disp('<< end of error message dump >>');
      | disp('------------------------------------------------------------');
      | disp(' ');
      | %Standard catch section END
      | end
      mask help: Setup one ADC channel.
      mask init:
      | %
      settings: CopyFcn=%deleted
      mask Help: web(which('IO_ADC.h'))
      mask Callback adc_channel: %
      mask Callback adc_type: %
      mask Callback range: %
      mask Callback pupd: %
      mask Callback sensor_supply: %
      mask Callback safety_conf: %
  ADC_Get : Subsystem  LoadFcn=|  mask(ADC_Get_Code){SampleTime=-1, ttlib=IO_Blk_Lib_TTC500, ttDescription=ADC_Get, tt_iolib_version=0.19, adc_channel=adc_channel}
      | try
      | %
      | %Upgrade Information - standard BEGIN
      | new_color = 'blue';
      | new_ver = '0.19';
      | act_ver = get_param(gcb,'tt_iolib_version');
      | if not(strcmp(act_ver,new_ver))
      |     disp(['Upgrade block: ',gcb,char(10),'       Version: ',act_ver,' -> ',new_ver]);
      |     %switch - case for specific upgrade information e.g. additional parameter required 
      |     %Change appearance and version information
      |     set_param(gcb,'ForegroundColor',new_color);
      |     set_param(gcb,'tt_iolib_version',new_ver);
      | end
      | %Upgrade Information - standard END
      | catch
      | %Standard catch section BEGIN 
      | disp(' ');
      | disp('------------------------------------------------------------');
      | disp('An error occurred in a callback of the TTC580-BlockLib.');
      | disp(['Please check the parameters in the mask of ',gcb]);
      | disp('If you do not encounter any violations, then please '); 
      | disp('copy the following lines and report this to support@ttcontrol.com ');
      | disp('<< begin of error message dump >>');
      | disp(['Version of TTC580-BlockLib: ', get_param(gcb,'tt_iolib_version')]);
      | disp(get_param(gcb,'ttDescription'));
      | disp(gcb);
      | x=lasterror;disp(x.message);
      | disp(get_param(gcb,'MaskValues'));
      | disp(version);
      | disp(computer);
      | disp('<< end of error message dump >>');
      | disp('------------------------------------------------------------');
      | disp(' ');
      | %Standard catch section END
      | end
      mask help: Returns the value of the given ADC channel.
      mask init:
      | %
      settings: CopyFcn=%deleted
      mask Help: web(which('IO_ADC.h'))
      mask Callback adc_channel: %
  PWM_Init : Terminator
  PWM_Init1 : Terminator
  ErrorCode : Outport  VectorParamsAs1DForOutWhenUnconnected=off
  adc_value : Outport  Port=2  VectorParamsAs1DForOutWhenUnconnected=off
  wires:
  ADC_ChannelInit/1(ErrorCode) -> PWM_Init/1
  ADC_Get/3(fresh) -> PWM_Init1/1
  ADC_Get/1(ErrorCode) -> ErrorCode/1
  ADC_Get/2(adc_value) -> adc_value/1
